simulink model "crc_syndrom"  (R2023b)
settings: Solver=VariableStepAuto  StartTime=0.0  StopTime=12  RelTol=1e-3
libraries: simulink_extras x5, simulink x1, hdlsllib x1
settings Model: Creator=user  LastModifiedBy=Mr_Dusza
settings SolverCC: AlgebraicLoopSolver=TrustRegion
settings DebuggingCC: UnconnectedInputMsg=warning  UnconnectedOutputMsg=warning  UnconnectedLineMsg=warning
settings ModelReferenceCC: EnableRefExpFcnMdlSchedulingChecks=on
settings SFSimCC: CustomCodeUndefinedFunction=UseInterfaceOnly

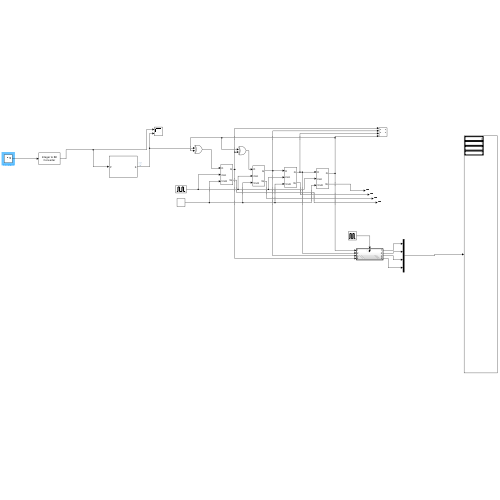
[thumbnail: Simulink's stored preview of the top-level diagram]
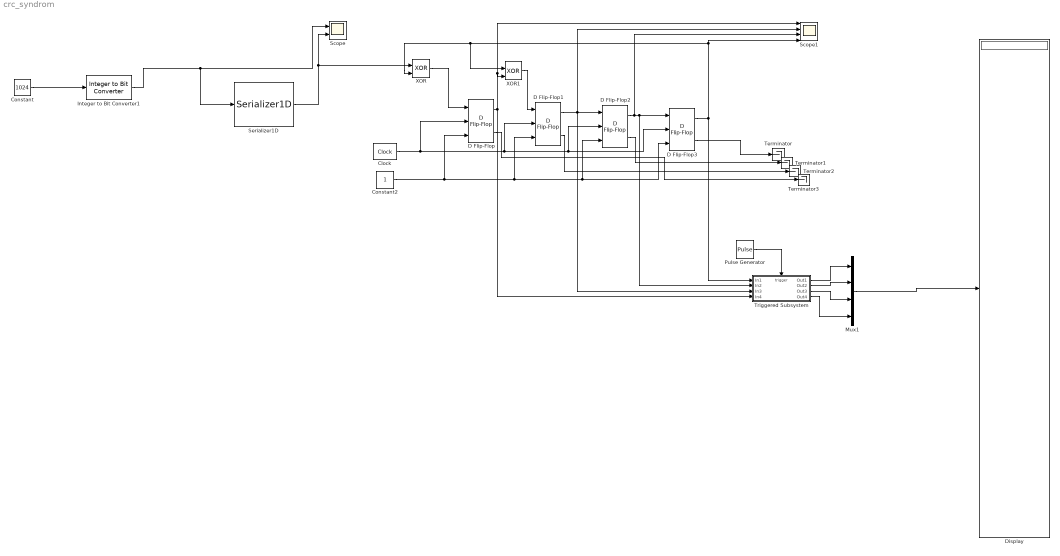
== system crc_syndrom ==
  Clock : simulink_extras/Flip Flops/Clock  period=1
  Constant : Constant  Value=1024
  Constant2 : Constant
  D Flip-Flop{,1..3} (4 alike) : simulink_extras/Flip Flops/D Flip-Flop
  Display : Display
      settings: Decimation=4
  Integer to Bit Converter1 : simulink/Logic and Bit Operations/Integer to Bit Converter  nbits=11  signedInputValues=Unsigned  bitOrder=MSB first  outDtype=boolean
      settings: LibrarySourceBlock=|
      | commutil2/Integer to Bit
      | Converter
  Mux1 : Mux
  Pulse Generator : DiscretePulseGenerator  PulseType=Time based  Period=1  PulseWidth=5  PhaseDelay=11.5
  Scope : Scope  NumInputPorts=2
  Scope1 : Scope  NumInputPorts=4
  Serializer1D : hdlsllib/HDL Operations/Serializer1D  Ratio=11  IdleCycles=0  validIn=off  startOut=off  validOut=off  inputDataDimensions=-1  inputSampleTime=11  inputSignalType=auto
  Terminator{,1..3} (4 alike) : Terminator
  Triggered Subsystem : Subsystem  TreatAsAtomicUnit=on
  XOR : Logic  Operator=XOR  IconShape=distinctive  AllPortsSameDT=off  OutDataTypeStr=boolean
  XOR1 : Logic  Operator=XOR  IconShape=distinctive  AllPortsSameDT=off  OutDataTypeStr=boolean
  wires:
  Constant/1 -> Integer to Bit Converter1/1
  Serializer1D/1 -> Scope/2, XOR/1
  XOR/1 -> D Flip-Flop/1
  D Flip-Flop1/1 -> Scope1/2, Triggered Subsystem/3(In3), D Flip-Flop2/1
  D Flip-Flop2/1 -> Triggered Subsystem/2(In2), D Flip-Flop3/1, Scope1/3
  D Flip-Flop/1 -> Triggered Subsystem/4(In4), Scope1/1, XOR1/2
  XOR1/1 -> D Flip-Flop1/1
  D Flip-Flop3/1 -> Triggered Subsystem/1(In1), Scope1/4, XOR1/1, XOR/2
  Constant2/1 -> D Flip-Flop/3, D Flip-Flop1/3, D Flip-Flop2/3, D Flip-Flop3/3
  Clock/1 -> D Flip-Flop/2, D Flip-Flop1/2, D Flip-Flop2/2, D Flip-Flop3/2
  Pulse Generator/1 -> Triggered Subsystem/Trigger
  D Flip-Flop3/2 -> Terminator/1
  D Flip-Flop2/2 -> Terminator1/1
  D Flip-Flop1/2 -> Terminator2/1
  D Flip-Flop/2 -> Terminator3/1
  Integer to Bit Converter1/1 -> Scope/1, Serializer1D/1
  Mux1/1 -> Display/1
  Triggered Subsystem/1(Out1) -> Mux1/1
  Triggered Subsystem/2(Out2) -> Mux1/2
  Triggered Subsystem/3(Out3) -> Mux1/3
  Triggered Subsystem/4(Out4) -> Mux1/4

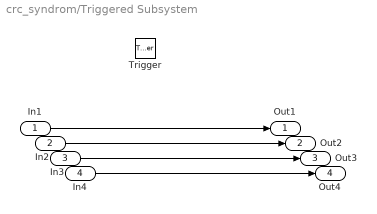
== system crc_syndrom/Triggered Subsystem ==
  In1 : Inport
  In2 : Inport  Port=2
  In3 : Inport  Port=3
  In4 : Inport  Port=4
  Trigger : TriggerPort  VariantControl=Variant
  Out1 : Outport  VectorParamsAs1DForOutWhenUnconnected=off
  Out2 : Outport  Port=2  VectorParamsAs1DForOutWhenUnconnected=off
  Out3 : Outport  Port=3  VectorParamsAs1DForOutWhenUnconnected=off
  Out4 : Outport  Port=4  VectorParamsAs1DForOutWhenUnconnected=off
  wires:
  In1/1 -> Out1/1
  In2/1 -> Out2/1
  In3/1 -> Out3/1
  In4/1 -> Out4/1
